simulink model "Assem1"  (R2017b)
settings: Solver=FixedStepAuto  StartTime=0.0  StopTime=40  FixedStep=0.01  RelTol=1e-3
model workspace: external: MATLAB File E:\RIC LAP Mo Phong\Robot4bac\Assem1_DataFile.m (data not in the file)
undefined symbols (not defined in the file or in its folder): smiData, X, Y, Z
libraries: sm_lib x29, nesl_utility x9, aerolibanimutils x1
settings Model: Creator=DELL  LastModifiedBy=DELL
settings OptimizationCC: BlockReduction=off

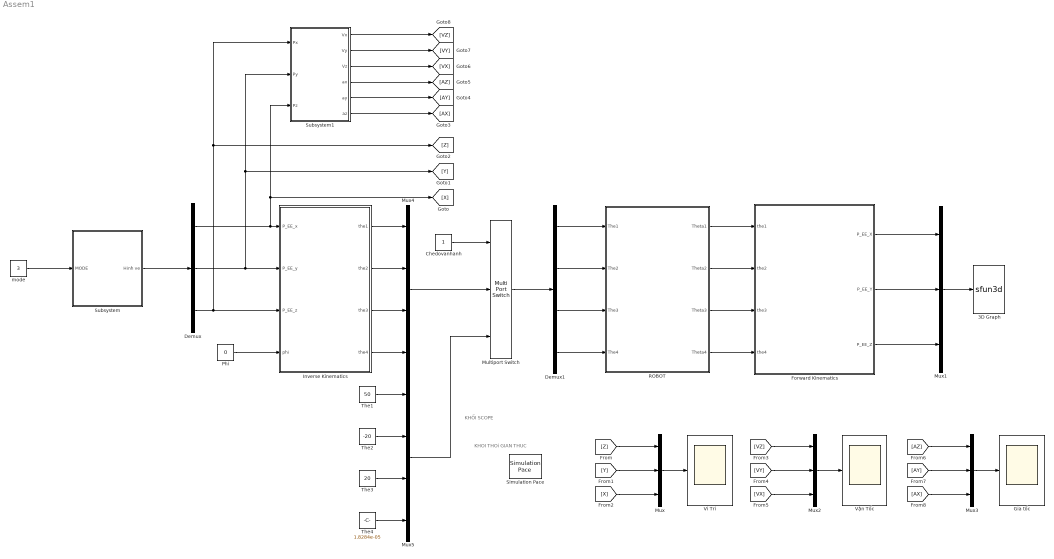
== system Assem1 ==
  note: KHOI THOi GIAN THUC
  note: KHỐI SCOPE
  3D Graph : S-Function  LoadFcn=if exist('sfun3d','file'), sfun3d([],[],[],'LoadBlock'); end  FunctionName=sfun3d  Parameters=ax,T,np,cp,gd,ls,mk,mx,hd,tb  SFunctionDeploymentMode=off  EnableBusSupport=off  mask(3D Graph){np=1, ax=[-500 1000 -500 1000 -500 1000], mx=1e4, T=0.01, cp=[3 2 1], gd=on, hd=off, tb=off, ls=:, mk=.}
      mask prompts: np "Number of moving points (lines)"; ax "Range: [xmin xmax  ymin ymax zmin zmax]"; mx "Max number of points in each line"; T "Sampling Time"; cp "Camera position (use [0 0 1] for 2D XY view)"; gd "Grid (on|off)"; hd "HeadMarkers (on|off)"; tb "Toolbar (on|off)"; ls "LineStyle"; mk "LineMarker"
      mask help:
      | This block plots the position of several points in the XYZ space. The input contains the coordinates of all the points (x1,y1,z1,x2,y2,z2,...).
      | The number of moving points (lines), the XYZ ranges, sampling time, camera position, and grid (among other things) can be set as mask parameters.
      settings: CopyFcn=if exist('sfun3d','file'), sfun3d([],[],[],'CopyBlock'); end  DeleteFcn=if exist('sfun3d','file'), sfun3d([],[],[],'DeleteBlock'); end  NameChangeFcn=if exist('sfun3d','file'), sfun3d([],[],[],'NameChange'); end
      mask Help:
      | This block plots the position of several points in the XYZ space. The input contains the coordinates of all the points (x1,y1,z1,x2,y2,z2,...).
      | The number of moving points (lines), the XYZ ranges, sampling time, camera position, and grid (among other things) can be set as mask parameters.
      mask TypeOptions ls: - | -- | : | -. | none
      mask TypeOptions mk: none | . | + | o | * | x | square | diamond | v | ^ | > | < | pentagram | hexagram
      mask Display: plot([.05 .95 .95 .05 .05],[.45 .45 .95 .95 .45], 0.5+cos(0:0.1:2*pi)*0.3,0.7+sin(0:0.1:2*pi)*0.2)
  Chedovanhanh : Constant
  Demux : Demux  Outputs=3
  Demux1 : Demux
  Forward Kinematics : MATLAB Function  TreatAsAtomicUnit=on
  Gia tốc : Scope
  Inverse Kinematics : MATLAB Function  TreatAsAtomicUnit=on
  Multiport Switch : MultiPortSwitch  Inputs=2
  Mux{,1..3} (4 alike) : Mux  Inputs=3
  Mux4 : Mux
  Mux5 : Mux
  Phi : Constant  Value=0
  "ROBOT " : Subsystem
  Simulation Pace : aerolibanimutils/Simulation Pace  SimulationPace=1  SleepMode=MATLAB Thread  OutputPaceError=off  SampleTime=0.01
  Subsystem : Subsystem
  Subsystem1 : Subsystem
  The1 : Constant  Value=50
  The2 : Constant  Value=-20
  The3 : Constant  Value=20
  The4 : Constant  Value=1.8284e-05
  Vi Tri : Scope
  Vận Tốc : Scope
  mode : Constant  Value=3
  wires:
  "ROBOT "/1(Theta1) -> Forward Kinematics/1(the1)
  "ROBOT "/2(Theta2) -> Forward Kinematics/2(the2)
  "ROBOT "/3(Theta3) -> Forward Kinematics/3(the3)
  "ROBOT "/4(Theta4) -> Forward Kinematics/4(the4)
  Chedovanhanh/1 -> Multiport Switch/1
  Mux4/1 -> Multiport Switch/2
  Multiport Switch/1 -> Demux1/1
  Inverse Kinematics/1(the1) -> Mux4/1
  Inverse Kinematics/2(the2) -> Mux4/2
  Inverse Kinematics/3(the3) -> Mux4/3
  Inverse Kinematics/4(the4) -> Mux4/4
  Demux1/1 -> "ROBOT "/1(The1)
  Demux1/2 -> "ROBOT "/2(The2)
  Demux1/3 -> "ROBOT "/3(The3)
  Demux1/4 -> "ROBOT "/4(The4)
  The4/1 -> Mux5/4
  The3/1 -> Mux5/3
  Mux5/1 -> Multiport Switch/3
  The1/1 -> Mux5/1
  The2/1 -> Mux5/2
  Subsystem/1(Hinh ve) -> Demux/1
  Subsystem1/3(Vz) -> [VX]
  Demux/3 -> Inverse Kinematics/3(P_EE_z), Subsystem1/1(Px), [Z]
  Subsystem1/6(az) -> [AX]
  Demux/2 -> Subsystem1/2(Py), [Y], Inverse Kinematics/2(P_EE_y)
  Subsystem1/2(Vy) -> [VY]
  Subsystem1/4(ax) -> [AZ]
  Subsystem1/5(ay) -> [AY]
  Subsystem1/1(Vx) -> [VZ]
  Demux/1 -> Subsystem1/3(Pz), [X], Inverse Kinematics/1(P_EE_x)
  [VY] -> Mux2/2
  Mux3/1 -> Gia tốc/1
  [VX] -> Mux2/3
  [AZ] -> Mux3/1
  [AY] -> Mux3/2
  Mux2/1 -> Vận Tốc/1
  [VZ] -> Mux2/1
  Mux/1 -> Vi Tri/1
  [Z] -> Mux/1
  [AX] -> Mux3/3
  [X] -> Mux/3
  [Y] -> Mux/2
  Mux1/1 -> 3D Graph/1
  Forward Kinematics/2(P_EE_Y) -> Mux1/2
  Forward Kinematics/3(P_EE_Z) -> Mux1/3
  Forward Kinematics/1(P_EE_X) -> Mux1/1
  mode/1 -> Subsystem/1(MODE)
  Phi/1 -> Inverse Kinematics/4(phi)

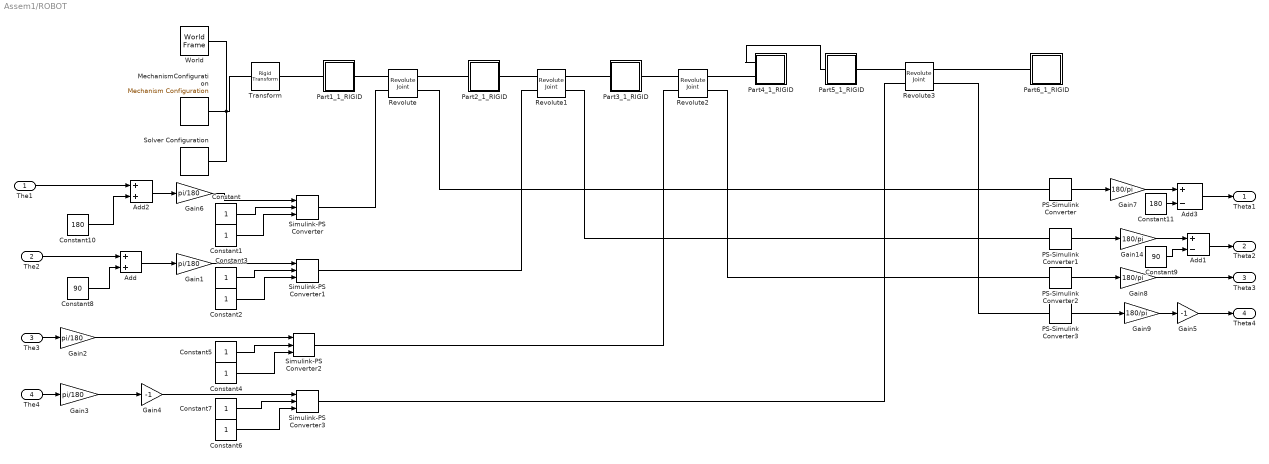
== system Assem1/ROBOT  ==
  The1 : Inport
  The2 : Inport  Port=2
  The3 : Inport  Port=3
  The4 : Inport  Port=4
  Add : Sum
  Add1 : Sum  Inputs=+-
  Add2 : Sum
  Add3 : Sum  Inputs=+-
  Constant{,1..7} (8 alike) : Constant
  Constant10 : Constant  Value=180
  Constant11 : Constant  Value=180
  Constant8 : Constant  Value=90
  Constant9 : Constant  Value=90
  Gain{1..3,6} (4 alike) : Gain  Gain=pi/180
  Gain{7..9,14} (4 alike) : Gain  Gain=180/pi
  Gain4 : Gain  Gain=-1
  Gain5 : Gain  Gain=-1
  MechanismConfiguration : sm_lib/Utilities/Mechanism Configuration  UniformGravity=Constant  GravityVector=[0 -9.80665 0]  GravityUnits=m/s^2  LinearizationDelta=0.001
  PS-Simulink Converter{,1..3} (4 alike) : nesl_utility/PS-Simulink Converter  PhysicalDomain=network_engine_domain  SubClassName=ps_output  LeftPortType=input  RightPortType=output  PseudoPeriodic=off  Frequencies=[]  Unit=1  AffineConversion=off
  Part1_1_RIGID : Subsystem
  Part2_1_RIGID : Subsystem
  Part3_1_RIGID : Subsystem
  Part4_1_RIGID : Subsystem
  Part5_1_RIGID : Subsystem
  Part6_1_RIGID : Subsystem
  Revolute : sm_lib/Joints/Revolute Joint  SenseConstraintForce=off  SenseConstraintForceX=off  SenseConstraintForceY=off  SenseConstraintForceZ=off  SenseConstraintTorque=off  SenseConstraintTorqueX=off  SenseConstraintTorqueY=off  SenseConstraintTorqueZ=off  SenseTotalForce=off  SenseTotalForceX=off  SenseTotalForceY=off  SenseTotalForceZ=off  SenseTotalTorque=off  SenseTotalTorqueX=off  SenseTotalTorqueY=off  SenseTotalTorqueZ=off  CompositeWrenchDir=FollowerOnBase  CompositeWrenchFrame=BaseFrame  EquilibriumPosition=0  EquilibriumPositionUnits=rad  SpringStiffness=0  SpringStiffnessUnits=N*m/rad  DampingCoefficient=0  DampingCoefficientUnits=N*m/(rad/s)  TorqueActuationMode=ComputedTorque  MotionActuationMode=InputMotion  SensePosition=on  SenseVelocity=off  SenseAcceleration=off  SenseTorqueForce=off  PositionTargetSpecify=on  PositionTargetPriority=Low  PositionTargetValue=smiData.RevoluteJoint(1).Rz.Pos  PositionTargetValueUnits=deg  VelocityTargetSpecify=off  VelocityTargetPriority=High  VelocityTargetValue=0  VelocityTargetValueUnits=deg/s
  Revolute1 : sm_lib/Joints/Revolute Joint  SenseConstraintForce=off  SenseConstraintForceX=off  SenseConstraintForceY=off  SenseConstraintForceZ=off  SenseConstraintTorque=off  SenseConstraintTorqueX=off  SenseConstraintTorqueY=off  SenseConstraintTorqueZ=off  SenseTotalForce=off  SenseTotalForceX=off  SenseTotalForceY=off  SenseTotalForceZ=off  SenseTotalTorque=off  SenseTotalTorqueX=off  SenseTotalTorqueY=off  SenseTotalTorqueZ=off  CompositeWrenchDir=FollowerOnBase  CompositeWrenchFrame=BaseFrame  EquilibriumPosition=0  EquilibriumPositionUnits=rad  SpringStiffness=0  SpringStiffnessUnits=N*m/rad  DampingCoefficient=0  DampingCoefficientUnits=N*m/(rad/s)  TorqueActuationMode=ComputedTorque  MotionActuationMode=InputMotion  SensePosition=on  SenseVelocity=off  SenseAcceleration=off  SenseTorqueForce=off  PositionTargetSpecify=on  PositionTargetPriority=Low  PositionTargetValue=smiData.RevoluteJoint(2).Rz.Pos  PositionTargetValueUnits=deg  VelocityTargetSpecify=off  VelocityTargetPriority=High  VelocityTargetValue=0  VelocityTargetValueUnits=deg/s
  Revolute2 : sm_lib/Joints/Revolute Joint  SenseConstraintForce=off  SenseConstraintForceX=off  SenseConstraintForceY=off  SenseConstraintForceZ=off  SenseConstraintTorque=off  SenseConstraintTorqueX=off  SenseConstraintTorqueY=off  SenseConstraintTorqueZ=off  SenseTotalForce=off  SenseTotalForceX=off  SenseTotalForceY=off  SenseTotalForceZ=off  SenseTotalTorque=off  SenseTotalTorqueX=off  SenseTotalTorqueY=off  SenseTotalTorqueZ=off  CompositeWrenchDir=FollowerOnBase  CompositeWrenchFrame=BaseFrame  EquilibriumPosition=0  EquilibriumPositionUnits=rad  SpringStiffness=0  SpringStiffnessUnits=N*m/rad  DampingCoefficient=0  DampingCoefficientUnits=N*m/(rad/s)  TorqueActuationMode=ComputedTorque  MotionActuationMode=InputMotion  SensePosition=on  SenseVelocity=off  SenseAcceleration=off  SenseTorqueForce=off  PositionTargetSpecify=on  PositionTargetPriority=Low  PositionTargetValue=smiData.RevoluteJoint(3).Rz.Pos  PositionTargetValueUnits=deg  VelocityTargetSpecify=off  VelocityTargetPriority=High  VelocityTargetValue=0  VelocityTargetValueUnits=deg/s
  Revolute3 : sm_lib/Joints/Revolute Joint  SenseConstraintForce=off  SenseConstraintForceX=off  SenseConstraintForceY=off  SenseConstraintForceZ=off  SenseConstraintTorque=off  SenseConstraintTorqueX=off  SenseConstraintTorqueY=off  SenseConstraintTorqueZ=off  SenseTotalForce=off  SenseTotalForceX=off  SenseTotalForceY=off  SenseTotalForceZ=off  SenseTotalTorque=off  SenseTotalTorqueX=off  SenseTotalTorqueY=off  SenseTotalTorqueZ=off  CompositeWrenchDir=FollowerOnBase  CompositeWrenchFrame=BaseFrame  EquilibriumPosition=0  EquilibriumPositionUnits=rad  SpringStiffness=0  SpringStiffnessUnits=N*m/rad  DampingCoefficient=0  DampingCoefficientUnits=N*m/(rad/s)  TorqueActuationMode=ComputedTorque  MotionActuationMode=InputMotion  SensePosition=on  SenseVelocity=off  SenseAcceleration=off  SenseTorqueForce=off  PositionTargetSpecify=on  PositionTargetPriority=Low  PositionTargetValue=smiData.RevoluteJoint(4).Rz.Pos  PositionTargetValueUnits=deg  VelocityTargetSpecify=off  VelocityTargetPriority=High  VelocityTargetValue=0  VelocityTargetValueUnits=deg/s
  Simulink-PS Converter{,1..3} (4 alike) : nesl_utility/Simulink-PS Converter  PhysicalDomain=network_engine_domain  SubClassName=ps_input  LeftPortType=input  RightPortType=output  PseudoPeriodic=off  Frequencies=[]  NoiseDistribution=none  NoiseParameters=[]  Unit=1  AffineConversion=off  FilteringAndDerivatives=provide  SimscapeFilterOrder=1  InputFilterTimeConstant=0.001  UdotUserProvided=2
  Solver Configuration : nesl_utility/Solver Configuration  PhysicalDomain=network_engine_domain  SubClassName=solver  LeftPortType=input  RightPortType=generic  Accelerate=off  Tones=[]  Harmonics=[]  SimulateNoise=off  Profile=off  UseLocalSampling=off  EnableSwitchedLinearOptims=on  FrequencyDomain=off  UseCCode=off  RelTol=0.001  AbsTol=1e-06  MinStep=1e-09  ToWorkspace=off  RevertToSquareIcSolve=off  NumHomotopyIterations=100  PhasorMode=off  PhasorModeNumHarmonics=1  DoDC=off  ResidualTolerance=1e-09  UseLocalSolver=off  LocalSolverChoice=NE_BACKWARD_EULER_ADVANCER  LocalSolverSampleTime=0.001  DoFixedCost=off  MaxNonlinIter=3  MaxModeIter=2  LinearAlgebra=Sparse  DelaysMemoryBudget=1024  AutomaticFiltering=on  FilteringTimeConstant=0.001
  Transform : sm_lib/Frames and Transforms/Rigid Transform  TranslationMethod=Cartesian  TranslationStandardOffset=0  TranslationLengthUnit=mm  TranslationStandardAxis=+Z  TranslationCartesianOffset=smiData.RigidTransform(11).translation  TranslationROffset=0  TranslationROffsetUnits=m  TranslationZOffset=0  TranslationZOffsetUnits=m  TranslationThetaOffset=0  TranslationThetaOffsetUnits=deg  RotationMethod=ArbitraryAxis  RotationAngleUnits=rad  RotationStandardAxis=+Z  RotationAngle=smiData.RigidTransform(11).angle  RotationArbitraryAxis=smiData.RigidTransform(11).axis  FollAlignAxisA=+X  BaseAlignAxisA=+Y  FollAlignAxisB=+Y  BaseAlignAxisB=+Z  RotationSequenceAxes=FollowerAxes  RotationSequence=XYX  RotationSequenceAngles=[0 0 0]  RotationSequenceAnglesUnits=deg  RotationMatrix=[1 0 0; 0 1 0; 0 0 1]
  World : sm_lib/Frames and Transforms/World Frame
  Theta1 : Outport
  Theta2 : Outport  Port=2
  Theta3 : Outport  Port=3
  Theta4 : Outport  Port=4
  wires:
  PS-Simulink Converter/1 -> Gain7/1
  PS-Simulink Converter3/1 -> Gain9/1
  Gain8/1 -> Theta3/1
  PS-Simulink Converter2/1 -> Gain8/1
  PS-Simulink Converter1/1 -> Gain14/1
  Gain2/1 -> Simulink-PS Converter2/1
  The3/1 -> Gain2/1
  Gain1/1 -> Simulink-PS Converter1/1
  Gain3/1 -> Gain4/1
  The4/1 -> Gain3/1
  Constant/1 -> Simulink-PS Converter/2
  Constant1/1 -> Simulink-PS Converter/3
  Constant3/1 -> Simulink-PS Converter1/2
  Constant2/1 -> Simulink-PS Converter1/3
  Constant5/1 -> Simulink-PS Converter2/2
  Constant4/1 -> Simulink-PS Converter2/3
  Constant7/1 -> Simulink-PS Converter3/2
  Constant6/1 -> Simulink-PS Converter3/3
  The2/1 -> Add/1
  Add/1 -> Gain1/1
  Constant8/1 -> Add/2
  Gain4/1 -> Simulink-PS Converter3/1
  Gain5/1 -> Theta4/1
  Gain9/1 -> Gain5/1
  Gain14/1 -> Add1/1
  Add1/1 -> Theta2/1
  Constant9/1 -> Add1/2
  Add2/1 -> Gain6/1
  Constant10/1 -> Add2/2
  Gain6/1 -> Simulink-PS Converter/1
  The1/1 -> Add2/1
  Gain7/1 -> Add3/1
  Add3/1 -> Theta1/1
  Constant11/1 -> Add3/2
  connections:
  PS-Simulink Converter/LConn1 -- Revolute/RConn2
  PS-Simulink Converter2/LConn1 -- Revolute2/RConn2
  PS-Simulink Converter1/LConn1 -- Revolute1/RConn2
  PS-Simulink Converter3/LConn1 -- Revolute3/RConn2
  Part2_1_RIGID/RConn1 -- Revolute1/LConn1
  Part2_1_RIGID/LConn1 -- Revolute/RConn1
  Part1_1_RIGID/LConn1 -- Transform/RConn1
  Part6_1_RIGID/LConn1 -- Revolute3/RConn1
  Part3_1_RIGID/LConn1 -- Revolute1/RConn1
  Part4_1_RIGID/LConn2 -- Revolute2/RConn1
  Part5_1_RIGID/RConn1 -- Revolute3/LConn1
  Part4_1_RIGID/LConn1 -- Part5_1_RIGID/LConn1
  Part3_1_RIGID/RConn1 -- Revolute2/LConn1
  Part1_1_RIGID/RConn1 -- Revolute/LConn1
  Transform/LConn1 -- MechanismConfiguration/RConn1 -- Solver Configuration/RConn1 -- World/RConn1
  Simulink-PS Converter/RConn1 -- Revolute/LConn2
  Simulink-PS Converter1/RConn1 -- Revolute1/LConn2
  Simulink-PS Converter3/RConn1 -- Revolute3/LConn2
  Simulink-PS Converter2/RConn1 -- Revolute2/LConn2

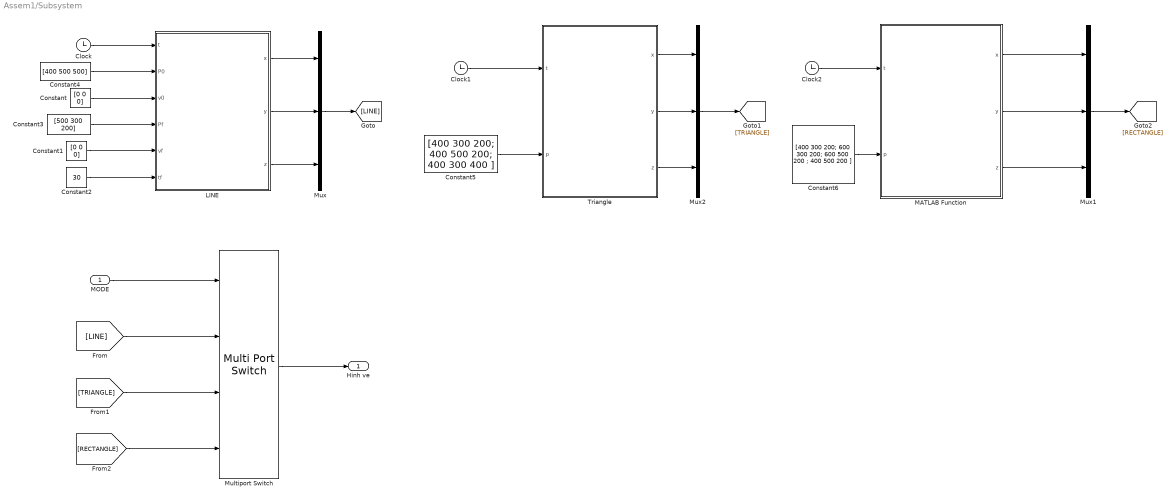
== system Assem1/Subsystem ==
  MODE : Inport
  Clock : Clock
      settings: Decimation=30
  Clock1 : Clock
      settings: Decimation=30
  Clock2 : Clock
      settings: Decimation=40
  Constant : Constant  Value=[0 0 0]
  Constant1 : Constant  Value=[0 0 0]
  Constant2 : Constant  Value=30
  Constant3 : Constant  Value=[500 300 200]
  Constant4 : Constant  Value=[400 500 500]
  Constant5 : Constant  Value="[400 300 200; 400 500 200; 400 300 400  ]"
  Constant6 : Constant  Value=[400 300 200; 600 300 200; 600 500 200 ; 400 500 200 ]
  "LINE   " : MATLAB Function  TreatAsAtomicUnit=on
  MATLAB Function : MATLAB Function  TreatAsAtomicUnit=on
  Multiport Switch : MultiPortSwitch
  Mux : Mux  Inputs=3
  Mux1 : Mux  Inputs=3
  Mux2 : Mux  Inputs=3
  Triangle : MATLAB Function  TreatAsAtomicUnit=on
  Hinh ve : Outport
  wires:
  Clock1/1 -> Triangle/1(t)
  Constant4/1 -> "LINE   "/2(P0)
  Constant3/1 -> "LINE   "/4(Pf)
  Clock/1 -> "LINE   "/1(t)
  Constant2/1 -> "LINE   "/6(tf)
  Constant/1 -> "LINE   "/3(v0)
  Constant1/1 -> "LINE   "/5(vf)
  MODE/1 -> Multiport Switch/1
  "LINE   "/1(x) -> Mux/1
  "LINE   "/2(y) -> Mux/2
  "LINE   "/3(z) -> Mux/3
  Mux/1 -> [LINE]
  [LINE] -> Multiport Switch/2
  [TRIANGLE] -> Multiport Switch/3
  [RECTANGLE] -> Multiport Switch/4
  Triangle/1(x) -> Mux2/1
  Triangle/2(y) -> Mux2/2
  Mux2/1 -> [TRIANGLE]
  Triangle/3(z) -> Mux2/3
  Constant5/1 -> Triangle/2(p)
  Mux1/1 -> [RECTANGLE]
  MATLAB Function/1(x) -> Mux1/1
  MATLAB Function/2(y) -> Mux1/2
  MATLAB Function/3(z) -> Mux1/3
  Clock2/1 -> MATLAB Function/1(t)
  Constant6/1 -> MATLAB Function/2(p)
  Multiport Switch/1 -> Hinh ve/1

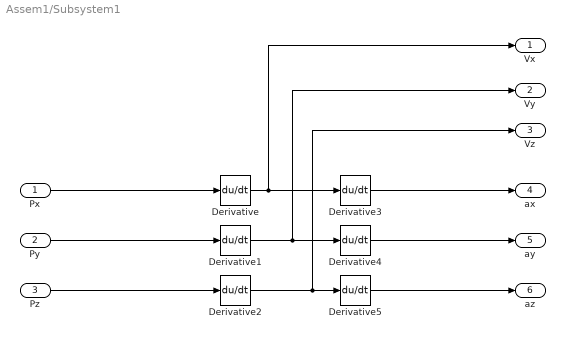
== system Assem1/Subsystem1 ==
  Px : Inport
  Py : Inport  Port=2
  Pz : Inport  Port=3
  Derivative{,1..5} (6 alike) : Derivative
  Vx : Outport
  Vy : Outport  Port=2
  Vz : Outport  Port=3
  ax : Outport  Port=4
  ay : Outport  Port=5
  az : Outport  Port=6
  wires:
  Derivative4/1 -> ay/1
  Px/1 -> Derivative/1
  Py/1 -> Derivative1/1
  Pz/1 -> Derivative2/1
  Derivative5/1 -> az/1
  Derivative2/1 -> Vz/1, Derivative5/1
  Derivative/1 -> Vx/1, Derivative3/1
  Derivative1/1 -> Vy/1, Derivative4/1
  Derivative3/1 -> ax/1

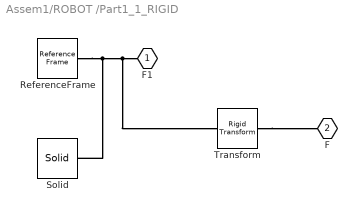
== system Assem1/ROBOT /Part1_1_RIGID ==
  ReferenceFrame : sm_lib/Frames and Transforms/Reference Frame
  Solid : sm_lib/Body Elements/Solid  InertiaType=Custom  Mass=smiData.Solid(4).mass  MassUnits=kg  CenterOfMass=smiData.Solid(4).CoM  CenterOfMassUnits=mm  MomentsOfInertia=smiData.Solid(4).MoI  MomentsOfInertiaUnits=kg*mm^2  ProductsOfInertia=smiData.Solid(4).PoI  ProductsOfInertiaUnits=kg*mm^2  DensityBased=on  Density=1000  DensityUnits=kg/m^3  DoExposeReferenceFrame=on  SerializedFrames=<Frames/>  GraphicType=FromGeometry  MarkerShape=Sphere  MarkerSize=10  GraphicVisPropType=SimpleVisualProperties  GraphicDiffuseColor=smiData.Solid(4).color  GraphicSpecularColor=[0.5 0.5 0.5 1.0]  GraphicAmbientColor=[0.15 0.15 0.15 1.0]  GraphicEmissiveColor=[0.0 0.0 0.0 1.0]  GraphicShininess=75  GraphicOpacity=smiData.Solid(4).opacity  GeometryShape=FromFile  RectangleSize=[1 1]  RectangleSizeUnits=m  BrickDimensions=[1 1 1]  BrickDimensionUnits=m  CylinderRadius=1  CylinderRadiusUnits=m  CylinderLength=1  CylinderLengthUnits=m  SphereRadius=1  SphereRadiusUnits=m  EllipsoidRadii=[1 1 1]  EllipsoidRadiiUnits=m  ExtrusionCrossSection=[1 1; -1 1; -1 -1; 1 -1]  ExtrusionCrossSectionUnits=m  ExtrusionLength=1  ExtrusionLengthUnits=m  PolygonNumSides=3  PolygonOuterRadius=1  PolygonOuterRadiusUnits=m  ExtGeomFileType=STEP  ExtGeomFileName=Part1_Default_sldprt.STEP  ExtGeomFileUnits=m  RevolutionCrossSection=[1 1; 1 -1; 2 -1; 2 1]  RevolutionCrossSectionUnits=m  RevolutionExtent=Full  RevolutionAngle=180  RevolutionAngleUnits=deg
  Transform : sm_lib/Frames and Transforms/Rigid Transform  TranslationMethod=Cartesian  TranslationStandardOffset=0  TranslationLengthUnit=mm  TranslationStandardAxis=+Z  TranslationCartesianOffset=smiData.RigidTransform(1).translation  TranslationROffset=0  TranslationROffsetUnits=m  TranslationZOffset=0  TranslationZOffsetUnits=m  TranslationThetaOffset=0  TranslationThetaOffsetUnits=deg  RotationMethod=ArbitraryAxis  RotationAngleUnits=rad  RotationStandardAxis=+Z  RotationAngle=smiData.RigidTransform(1).angle  RotationArbitraryAxis=smiData.RigidTransform(1).axis  FollAlignAxisA=+X  BaseAlignAxisA=+Y  FollAlignAxisB=+Y  BaseAlignAxisB=+Z  RotationSequenceAxes=FollowerAxes  RotationSequence=XYX  RotationSequenceAngles=[0 0 0]  RotationSequenceAnglesUnits=deg  RotationMatrix=[1 0 0; 0 1 0; 0 0 1]
  F1 : PMIOPort  Port=1  Side=Left
  F : PMIOPort  Port=2  Side=Right
  connections:
  Solid/RConn1 -- ReferenceFrame/RConn1 -- Transform/LConn1 -- F1/RConn1
  Transform/RConn1 -- F/RConn1

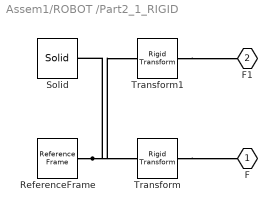
== system Assem1/ROBOT /Part2_1_RIGID ==
  ReferenceFrame : sm_lib/Frames and Transforms/Reference Frame
  Solid : sm_lib/Body Elements/Solid  InertiaType=Custom  Mass=smiData.Solid(2).mass  MassUnits=kg  CenterOfMass=smiData.Solid(2).CoM  CenterOfMassUnits=mm  MomentsOfInertia=smiData.Solid(2).MoI  MomentsOfInertiaUnits=kg*mm^2  ProductsOfInertia=smiData.Solid(2).PoI  ProductsOfInertiaUnits=kg*mm^2  DensityBased=on  Density=1000  DensityUnits=kg/m^3  DoExposeReferenceFrame=on  SerializedFrames=<Frames/>  GraphicType=FromGeometry  MarkerShape=Sphere  MarkerSize=10  GraphicVisPropType=SimpleVisualProperties  GraphicDiffuseColor=smiData.Solid(2).color  GraphicSpecularColor=[0.5 0.5 0.5 1.0]  GraphicAmbientColor=[0.15 0.15 0.15 1.0]  GraphicEmissiveColor=[0.0 0.0 0.0 1.0]  GraphicShininess=75  GraphicOpacity=smiData.Solid(2).opacity  GeometryShape=FromFile  RectangleSize=[1 1]  RectangleSizeUnits=m  BrickDimensions=[1 1 1]  BrickDimensionUnits=m  CylinderRadius=1  CylinderRadiusUnits=m  CylinderLength=1  CylinderLengthUnits=m  SphereRadius=1  SphereRadiusUnits=m  EllipsoidRadii=[1 1 1]  EllipsoidRadiiUnits=m  ExtrusionCrossSection=[1 1; -1 1; -1 -1; 1 -1]  ExtrusionCrossSectionUnits=m  ExtrusionLength=1  ExtrusionLengthUnits=m  PolygonNumSides=3  PolygonOuterRadius=1  PolygonOuterRadiusUnits=m  ExtGeomFileType=STEP  ExtGeomFileName=Part2_Default_sldprt.STEP  ExtGeomFileUnits=m  RevolutionCrossSection=[1 1; 1 -1; 2 -1; 2 1]  RevolutionCrossSectionUnits=m  RevolutionExtent=Full  RevolutionAngle=180  RevolutionAngleUnits=deg
  Transform : sm_lib/Frames and Transforms/Rigid Transform  TranslationMethod=Cartesian  TranslationStandardOffset=0  TranslationLengthUnit=mm  TranslationStandardAxis=+Z  TranslationCartesianOffset=smiData.RigidTransform(2).translation  TranslationROffset=0  TranslationROffsetUnits=m  TranslationZOffset=0  TranslationZOffsetUnits=m  TranslationThetaOffset=0  TranslationThetaOffsetUnits=deg  RotationMethod=ArbitraryAxis  RotationAngleUnits=rad  RotationStandardAxis=+Z  RotationAngle=smiData.RigidTransform(2).angle  RotationArbitraryAxis=smiData.RigidTransform(2).axis  FollAlignAxisA=+X  BaseAlignAxisA=+Y  FollAlignAxisB=+Y  BaseAlignAxisB=+Z  RotationSequenceAxes=FollowerAxes  RotationSequence=XYX  RotationSequenceAngles=[0 0 0]  RotationSequenceAnglesUnits=deg  RotationMatrix=[1 0 0; 0 1 0; 0 0 1]
  Transform1 : sm_lib/Frames and Transforms/Rigid Transform  TranslationMethod=Cartesian  TranslationStandardOffset=0  TranslationLengthUnit=mm  TranslationStandardAxis=+Z  TranslationCartesianOffset=smiData.RigidTransform(3).translation  TranslationROffset=0  TranslationROffsetUnits=m  TranslationZOffset=0  TranslationZOffsetUnits=m  TranslationThetaOffset=0  TranslationThetaOffsetUnits=deg  RotationMethod=ArbitraryAxis  RotationAngleUnits=rad  RotationStandardAxis=+Z  RotationAngle=smiData.RigidTransform(3).angle  RotationArbitraryAxis=smiData.RigidTransform(3).axis  FollAlignAxisA=+X  BaseAlignAxisA=+Y  FollAlignAxisB=+Y  BaseAlignAxisB=+Z  RotationSequenceAxes=FollowerAxes  RotationSequence=XYX  RotationSequenceAngles=[0 0 0]  RotationSequenceAnglesUnits=deg  RotationMatrix=[1 0 0; 0 1 0; 0 0 1]
  F : PMIOPort  Port=1  Side=Left
  F1 : PMIOPort  Port=2  Side=Right
  connections:
  Solid/RConn1 -- ReferenceFrame/RConn1 -- Transform/LConn1 -- Transform1/LConn1
  Transform/RConn1 -- F/RConn1
  Transform1/RConn1 -- F1/RConn1

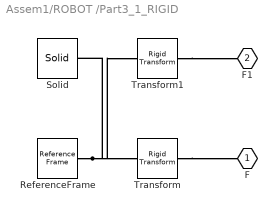
== system Assem1/ROBOT /Part3_1_RIGID ==
  ReferenceFrame : sm_lib/Frames and Transforms/Reference Frame
  Solid : sm_lib/Body Elements/Solid  InertiaType=Custom  Mass=smiData.Solid(3).mass  MassUnits=kg  CenterOfMass=smiData.Solid(3).CoM  CenterOfMassUnits=mm  MomentsOfInertia=smiData.Solid(3).MoI  MomentsOfInertiaUnits=kg*mm^2  ProductsOfInertia=smiData.Solid(3).PoI  ProductsOfInertiaUnits=kg*mm^2  DensityBased=on  Density=1000  DensityUnits=kg/m^3  DoExposeReferenceFrame=on  SerializedFrames=<Frames/>  GraphicType=FromGeometry  MarkerShape=Sphere  MarkerSize=10  GraphicVisPropType=SimpleVisualProperties  GraphicDiffuseColor=smiData.Solid(3).color  GraphicSpecularColor=[0.5 0.5 0.5 1.0]  GraphicAmbientColor=[0.15 0.15 0.15 1.0]  GraphicEmissiveColor=[0.0 0.0 0.0 1.0]  GraphicShininess=75  GraphicOpacity=smiData.Solid(3).opacity  GeometryShape=FromFile  RectangleSize=[1 1]  RectangleSizeUnits=m  BrickDimensions=[1 1 1]  BrickDimensionUnits=m  CylinderRadius=1  CylinderRadiusUnits=m  CylinderLength=1  CylinderLengthUnits=m  SphereRadius=1  SphereRadiusUnits=m  EllipsoidRadii=[1 1 1]  EllipsoidRadiiUnits=m  ExtrusionCrossSection=[1 1; -1 1; -1 -1; 1 -1]  ExtrusionCrossSectionUnits=m  ExtrusionLength=1  ExtrusionLengthUnits=m  PolygonNumSides=3  PolygonOuterRadius=1  PolygonOuterRadiusUnits=m  ExtGeomFileType=STEP  ExtGeomFileName=Part3_Default_sldprt.STEP  ExtGeomFileUnits=m  RevolutionCrossSection=[1 1; 1 -1; 2 -1; 2 1]  RevolutionCrossSectionUnits=m  RevolutionExtent=Full  RevolutionAngle=180  RevolutionAngleUnits=deg
  Transform : sm_lib/Frames and Transforms/Rigid Transform  TranslationMethod=Cartesian  TranslationStandardOffset=0  TranslationLengthUnit=mm  TranslationStandardAxis=+Z  TranslationCartesianOffset=smiData.RigidTransform(4).translation  TranslationROffset=0  TranslationROffsetUnits=m  TranslationZOffset=0  TranslationZOffsetUnits=m  TranslationThetaOffset=0  TranslationThetaOffsetUnits=deg  RotationMethod=ArbitraryAxis  RotationAngleUnits=rad  RotationStandardAxis=+Z  RotationAngle=smiData.RigidTransform(4).angle  RotationArbitraryAxis=smiData.RigidTransform(4).axis  FollAlignAxisA=+X  BaseAlignAxisA=+Y  FollAlignAxisB=+Y  BaseAlignAxisB=+Z  RotationSequenceAxes=FollowerAxes  RotationSequence=XYX  RotationSequenceAngles=[0 0 0]  RotationSequenceAnglesUnits=deg  RotationMatrix=[1 0 0; 0 1 0; 0 0 1]
  Transform1 : sm_lib/Frames and Transforms/Rigid Transform  TranslationMethod=Cartesian  TranslationStandardOffset=0  TranslationLengthUnit=mm  TranslationStandardAxis=+Z  TranslationCartesianOffset=smiData.RigidTransform(5).translation  TranslationROffset=0  TranslationROffsetUnits=m  TranslationZOffset=0  TranslationZOffsetUnits=m  TranslationThetaOffset=0  TranslationThetaOffsetUnits=deg  RotationMethod=ArbitraryAxis  RotationAngleUnits=rad  RotationStandardAxis=+Z  RotationAngle=smiData.RigidTransform(5).angle  RotationArbitraryAxis=smiData.RigidTransform(5).axis  FollAlignAxisA=+X  BaseAlignAxisA=+Y  FollAlignAxisB=+Y  BaseAlignAxisB=+Z  RotationSequenceAxes=FollowerAxes  RotationSequence=XYX  RotationSequenceAngles=[0 0 0]  RotationSequenceAnglesUnits=deg  RotationMatrix=[1 0 0; 0 1 0; 0 0 1]
  F : PMIOPort  Port=1  Side=Left
  F1 : PMIOPort  Port=2  Side=Right
  connections:
  Solid/RConn1 -- ReferenceFrame/RConn1 -- Transform/LConn1 -- Transform1/LConn1
  Transform/RConn1 -- F/RConn1
  Transform1/RConn1 -- F1/RConn1

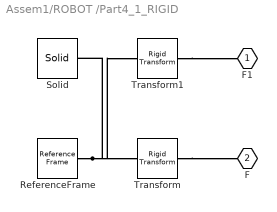
== system Assem1/ROBOT /Part4_1_RIGID ==
  ReferenceFrame : sm_lib/Frames and Transforms/Reference Frame
  Solid : sm_lib/Body Elements/Solid  InertiaType=Custom  Mass=smiData.Solid(1).mass  MassUnits=kg  CenterOfMass=smiData.Solid(1).CoM  CenterOfMassUnits=mm  MomentsOfInertia=smiData.Solid(1).MoI  MomentsOfInertiaUnits=kg*mm^2  ProductsOfInertia=smiData.Solid(1).PoI  ProductsOfInertiaUnits=kg*mm^2  DensityBased=on  Density=1000  DensityUnits=kg/m^3  DoExposeReferenceFrame=on  SerializedFrames=<Frames/>  GraphicType=FromGeometry  MarkerShape=Sphere  MarkerSize=10  GraphicVisPropType=SimpleVisualProperties  GraphicDiffuseColor=smiData.Solid(1).color  GraphicSpecularColor=[0.5 0.5 0.5 1.0]  GraphicAmbientColor=[0.15 0.15 0.15 1.0]  GraphicEmissiveColor=[0.0 0.0 0.0 1.0]  GraphicShininess=75  GraphicOpacity=smiData.Solid(1).opacity  GeometryShape=FromFile  RectangleSize=[1 1]  RectangleSizeUnits=m  BrickDimensions=[1 1 1]  BrickDimensionUnits=m  CylinderRadius=1  CylinderRadiusUnits=m  CylinderLength=1  CylinderLengthUnits=m  SphereRadius=1  SphereRadiusUnits=m  EllipsoidRadii=[1 1 1]  EllipsoidRadiiUnits=m  ExtrusionCrossSection=[1 1; -1 1; -1 -1; 1 -1]  ExtrusionCrossSectionUnits=m  ExtrusionLength=1  ExtrusionLengthUnits=m  PolygonNumSides=3  PolygonOuterRadius=1  PolygonOuterRadiusUnits=m  ExtGeomFileType=STEP  ExtGeomFileName=Part4_Default_sldprt.STEP  ExtGeomFileUnits=m  RevolutionCrossSection=[1 1; 1 -1; 2 -1; 2 1]  RevolutionCrossSectionUnits=m  RevolutionExtent=Full  RevolutionAngle=180  RevolutionAngleUnits=deg
  Transform : sm_lib/Frames and Transforms/Rigid Transform  TranslationMethod=Cartesian  TranslationStandardOffset=0  TranslationLengthUnit=mm  TranslationStandardAxis=+Z  TranslationCartesianOffset=smiData.RigidTransform(6).translation  TranslationROffset=0  TranslationROffsetUnits=m  TranslationZOffset=0  TranslationZOffsetUnits=m  TranslationThetaOffset=0  TranslationThetaOffsetUnits=deg  RotationMethod=ArbitraryAxis  RotationAngleUnits=rad  RotationStandardAxis=+Z  RotationAngle=smiData.RigidTransform(6).angle  RotationArbitraryAxis=smiData.RigidTransform(6).axis  FollAlignAxisA=+X  BaseAlignAxisA=+Y  FollAlignAxisB=+Y  BaseAlignAxisB=+Z  RotationSequenceAxes=FollowerAxes  RotationSequence=XYX  RotationSequenceAngles=[0 0 0]  RotationSequenceAnglesUnits=deg  RotationMatrix=[1 0 0; 0 1 0; 0 0 1]
  Transform1 : sm_lib/Frames and Transforms/Rigid Transform  TranslationMethod=Cartesian  TranslationStandardOffset=0  TranslationLengthUnit=mm  TranslationStandardAxis=+Z  TranslationCartesianOffset=smiData.RigidTransform(7).translation  TranslationROffset=0  TranslationROffsetUnits=m  TranslationZOffset=0  TranslationZOffsetUnits=m  TranslationThetaOffset=0  TranslationThetaOffsetUnits=deg  RotationMethod=ArbitraryAxis  RotationAngleUnits=rad  RotationStandardAxis=+Z  RotationAngle=smiData.RigidTransform(7).angle  RotationArbitraryAxis=smiData.RigidTransform(7).axis  FollAlignAxisA=+X  BaseAlignAxisA=+Y  FollAlignAxisB=+Y  BaseAlignAxisB=+Z  RotationSequenceAxes=FollowerAxes  RotationSequence=XYX  RotationSequenceAngles=[0 0 0]  RotationSequenceAnglesUnits=deg  RotationMatrix=[1 0 0; 0 1 0; 0 0 1]
  F1 : PMIOPort  Port=1  Side=Left
  F : PMIOPort  Port=2  Side=Left
  connections:
  Solid/RConn1 -- ReferenceFrame/RConn1 -- Transform/LConn1 -- Transform1/LConn1
  Transform/RConn1 -- F/RConn1
  Transform1/RConn1 -- F1/RConn1

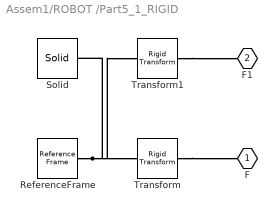
== system Assem1/ROBOT /Part5_1_RIGID ==
  ReferenceFrame : sm_lib/Frames and Transforms/Reference Frame
  Solid : sm_lib/Body Elements/Solid  InertiaType=Custom  Mass=smiData.Solid(6).mass  MassUnits=kg  CenterOfMass=smiData.Solid(6).CoM  CenterOfMassUnits=mm  MomentsOfInertia=smiData.Solid(6).MoI  MomentsOfInertiaUnits=kg*mm^2  ProductsOfInertia=smiData.Solid(6).PoI  ProductsOfInertiaUnits=kg*mm^2  DensityBased=on  Density=1000  DensityUnits=kg/m^3  DoExposeReferenceFrame=on  SerializedFrames=<Frames/>  GraphicType=FromGeometry  MarkerShape=Sphere  MarkerSize=10  GraphicVisPropType=SimpleVisualProperties  GraphicDiffuseColor=smiData.Solid(6).color  GraphicSpecularColor=[0.5 0.5 0.5 1.0]  GraphicAmbientColor=[0.15 0.15 0.15 1.0]  GraphicEmissiveColor=[0.0 0.0 0.0 1.0]  GraphicShininess=75  GraphicOpacity=smiData.Solid(6).opacity  GeometryShape=FromFile  RectangleSize=[1 1]  RectangleSizeUnits=m  BrickDimensions=[1 1 1]  BrickDimensionUnits=m  CylinderRadius=1  CylinderRadiusUnits=m  CylinderLength=1  CylinderLengthUnits=m  SphereRadius=1  SphereRadiusUnits=m  EllipsoidRadii=[1 1 1]  EllipsoidRadiiUnits=m  ExtrusionCrossSection=[1 1; -1 1; -1 -1; 1 -1]  ExtrusionCrossSectionUnits=m  ExtrusionLength=1  ExtrusionLengthUnits=m  PolygonNumSides=3  PolygonOuterRadius=1  PolygonOuterRadiusUnits=m  ExtGeomFileType=STEP  ExtGeomFileName=Part5_Default_sldprt.STEP  ExtGeomFileUnits=m  RevolutionCrossSection=[1 1; 1 -1; 2 -1; 2 1]  RevolutionCrossSectionUnits=m  RevolutionExtent=Full  RevolutionAngle=180  RevolutionAngleUnits=deg
  Transform : sm_lib/Frames and Transforms/Rigid Transform  TranslationMethod=Cartesian  TranslationStandardOffset=0  TranslationLengthUnit=mm  TranslationStandardAxis=+Z  TranslationCartesianOffset=smiData.RigidTransform(8).translation  TranslationROffset=0  TranslationROffsetUnits=m  TranslationZOffset=0  TranslationZOffsetUnits=m  TranslationThetaOffset=0  TranslationThetaOffsetUnits=deg  RotationMethod=ArbitraryAxis  RotationAngleUnits=rad  RotationStandardAxis=+Z  RotationAngle=smiData.RigidTransform(8).angle  RotationArbitraryAxis=smiData.RigidTransform(8).axis  FollAlignAxisA=+X  BaseAlignAxisA=+Y  FollAlignAxisB=+Y  BaseAlignAxisB=+Z  RotationSequenceAxes=FollowerAxes  RotationSequence=XYX  RotationSequenceAngles=[0 0 0]  RotationSequenceAnglesUnits=deg  RotationMatrix=[1 0 0; 0 1 0; 0 0 1]
  Transform1 : sm_lib/Frames and Transforms/Rigid Transform  TranslationMethod=Cartesian  TranslationStandardOffset=0  TranslationLengthUnit=mm  TranslationStandardAxis=+Z  TranslationCartesianOffset=smiData.RigidTransform(9).translation  TranslationROffset=0  TranslationROffsetUnits=m  TranslationZOffset=0  TranslationZOffsetUnits=m  TranslationThetaOffset=0  TranslationThetaOffsetUnits=deg  RotationMethod=ArbitraryAxis  RotationAngleUnits=rad  RotationStandardAxis=+Z  RotationAngle=smiData.RigidTransform(9).angle  RotationArbitraryAxis=smiData.RigidTransform(9).axis  FollAlignAxisA=+X  BaseAlignAxisA=+Y  FollAlignAxisB=+Y  BaseAlignAxisB=+Z  RotationSequenceAxes=FollowerAxes  RotationSequence=XYX  RotationSequenceAngles=[0 0 0]  RotationSequenceAnglesUnits=deg  RotationMatrix=[1 0 0; 0 1 0; 0 0 1]
  F : PMIOPort  Port=1  Side=Left
  F1 : PMIOPort  Port=2  Side=Right
  connections:
  Solid/RConn1 -- ReferenceFrame/RConn1 -- Transform/LConn1 -- Transform1/LConn1
  Transform/RConn1 -- F/RConn1
  Transform1/RConn1 -- F1/RConn1

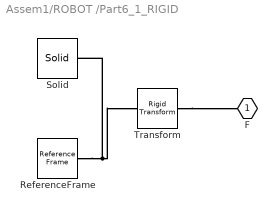
== system Assem1/ROBOT /Part6_1_RIGID ==
  ReferenceFrame : sm_lib/Frames and Transforms/Reference Frame
  Solid : sm_lib/Body Elements/Solid  InertiaType=Custom  Mass=smiData.Solid(5).mass  MassUnits=kg  CenterOfMass=smiData.Solid(5).CoM  CenterOfMassUnits=mm  MomentsOfInertia=smiData.Solid(5).MoI  MomentsOfInertiaUnits=kg*mm^2  ProductsOfInertia=smiData.Solid(5).PoI  ProductsOfInertiaUnits=kg*mm^2  DensityBased=on  Density=1000  DensityUnits=kg/m^3  DoExposeReferenceFrame=on  SerializedFrames=<Frames/>  GraphicType=FromGeometry  MarkerShape=Sphere  MarkerSize=10  GraphicVisPropType=SimpleVisualProperties  GraphicDiffuseColor=smiData.Solid(5).color  GraphicSpecularColor=[0.5 0.5 0.5 1.0]  GraphicAmbientColor=[0.15 0.15 0.15 1.0]  GraphicEmissiveColor=[0.0 0.0 0.0 1.0]  GraphicShininess=75  GraphicOpacity=smiData.Solid(5).opacity  GeometryShape=FromFile  RectangleSize=[1 1]  RectangleSizeUnits=m  BrickDimensions=[1 1 1]  BrickDimensionUnits=m  CylinderRadius=1  CylinderRadiusUnits=m  CylinderLength=1  CylinderLengthUnits=m  SphereRadius=1  SphereRadiusUnits=m  EllipsoidRadii=[1 1 1]  EllipsoidRadiiUnits=m  ExtrusionCrossSection=[1 1; -1 1; -1 -1; 1 -1]  ExtrusionCrossSectionUnits=m  ExtrusionLength=1  ExtrusionLengthUnits=m  PolygonNumSides=3  PolygonOuterRadius=1  PolygonOuterRadiusUnits=m  ExtGeomFileType=STEP  ExtGeomFileName=Part6_Default_sldprt.STEP  ExtGeomFileUnits=m  RevolutionCrossSection=[1 1; 1 -1; 2 -1; 2 1]  RevolutionCrossSectionUnits=m  RevolutionExtent=Full  RevolutionAngle=180  RevolutionAngleUnits=deg
  Transform : sm_lib/Frames and Transforms/Rigid Transform  TranslationMethod=Cartesian  TranslationStandardOffset=0  TranslationLengthUnit=mm  TranslationStandardAxis=+Z  TranslationCartesianOffset=smiData.RigidTransform(10).translation  TranslationROffset=0  TranslationROffsetUnits=m  TranslationZOffset=0  TranslationZOffsetUnits=m  TranslationThetaOffset=0  TranslationThetaOffsetUnits=deg  RotationMethod=ArbitraryAxis  RotationAngleUnits=rad  RotationStandardAxis=+Z  RotationAngle=smiData.RigidTransform(10).angle  RotationArbitraryAxis=smiData.RigidTransform(10).axis  FollAlignAxisA=+X  BaseAlignAxisA=+Y  FollAlignAxisB=+Y  BaseAlignAxisB=+Z  RotationSequenceAxes=FollowerAxes  RotationSequence=XYX  RotationSequenceAngles=[0 0 0]  RotationSequenceAnglesUnits=deg  RotationMatrix=[1 0 0; 0 1 0; 0 0 1]
  F : PMIOPort  Port=1  Side=Left
  connections:
  Solid/RConn1 -- ReferenceFrame/RConn1 -- Transform/LConn1
  Transform/RConn1 -- F/RConn1

== matlab function Assem1/Inverse Kinematics ==
  data: P_EE_x input; P_EE_y input; P_EE_z input; the1 output; phi input; the2 output; the3 output; the4 output
function [the1,the2,the3,the4]=IK_4DOF(P_EE_x,P_EE_y,P_EE_z,phi)
l1=150; l2=350; l3=363.5; l4=210;
d1=140;
 % tim the1
the1=atan2d(P_EE_y,P_EE_x);
Px=P_EE_x-l4*cosd(the1)*cosd(phi);
Py=P_EE_y-l4*sind(the1)*cosd(phi);
Pz=P_EE_z+l4*sind(phi);

 %tim theta3 >0
 nx=Px*cosd(the1)+Py*sind(the1)-l1;
 ny=Pz-d1;
 c3=(nx*nx+ny*ny-l3*l3-l2*l2)/(2*l2*l3);
 s3=sqrt(1-c3^2);
 the3=atan2d(s3,c3);
 %tim theta2 >0;
 the2=atan2d(-((ny*(l3*cosd(the3)+l2)+l3*sind(the3)*nx)),-((-nx*(l3*cosd(the3)+l2)+l3*sind(the3)*ny)));
 %tim theta4 
 the4=phi-the2-the3;

== matlab function Assem1/Forward Kinematics ==
  data: the1 input; P_EE_X output; the2 input; the3 input; the4 input; P_EE_Y output; P_EE_Z output
function [P_EE_X,P_EE_Y,P_EE_Z]=FK_4DOF(the1,the2,the3,the4)
l1=150; l2=350; l3=363.5; l4=210;
d1=140;
P_EE_X=cosd(the1)*(l1+l3*cosd(the2+the3)+l2*cosd(the2)+l4*cosd(the2+the3+the4));
P_EE_Y=sind(the1)*(l1+l3*cosd(the2+the3)+l2*cosd(the2)+l4*cosd(the2+the3+the4));
P_EE_Z=d1-l3*sind(the2+the3)-l2*sind(the2)-l4*sind(the2+the3+the4);
end

== matlab function Assem1/Subsystem/LINE    ==
  data: x output; t input; y output; P0 input; v0 input; Pf input; vf input; tf input; z output
function [x,y,z] = LINE(t,P0,v0,Pf,vf,tf)
a10=P0(1);
a20=P0(2);
a30=P0(3);
a11=v0(1);
a21=v0(2);
a31=v0(3);
a12=3/tf^2*(Pf(1)-P0(1))-2/tf*v0(1)-1/tf*vf(1);
a22=3/tf^2*(Pf(2)-P0(2))-2/tf*v0(2)-1/tf*vf(2);
a32=3/tf^2*(Pf(3)-P0(3))-2/tf*v0(3)-1/tf*vf(3);
a13=-2/tf^3*(Pf(1)-P0(1))+1/tf^2*(vf(1)+v0(1));
a23=-2/tf^3*(Pf(2)-P0(2))+1/tf^2*(vf(2)+v0(2));
a33=-2/tf^3*(Pf(3)-P0(3))+1/tf^2*(vf(3)+v0(3));
if t<30
    x=a10+a11*t+a12*t^2+a13*t^3;
    y=a20+a21*t+a22*t^2+a23*t^3;
    z=a30+a31*t+a32*t^2+a33*t^3; 
else
    t=30;
    x=a10+a11*t+a12*t^2+a13*t^3;
    y=a20+a21*t+a22*t^2+a23*t^3;
    z=a30+a31*t+a32*t^2+a33*t^3; 
end

== matlab function Assem1/Subsystem/Triangle ==
  data: x output; t input; y output; p input; z output
function [x,y,z] = Triangle(t,p)
t0=0;
tf=10;
t1=t;
v0=0;
vf=0;
%Phương trình quĩ đạo bậc 3: P(t) = a0 + a1*t+ a2*t^2 + a3*t^3
A=[ 1 t0 t0^2 t0^3;
    0  1  2*t0 3*t0^2; 
    1 tf tf^2 tf^3;
    0 1  2*tf 3*tf^2;];
if t<=10
%%
C=[ p(1,1); v0; p(2,1); vf];
Bx=A\C;
x = Bx(1,1) + Bx(2,1)*t1 +Bx(3,1)*t1^2 + Bx(4,1)*t1^3;
C=[p(1,2); v0; p(2,2); vf];
By=A\C;
y = By(1,1) + By(2,1)*t1 +By(3,1)*t1^2 + By(4,1)*t1^3;
C=[p(1,3); v0; p(2,3); vf];
Bz=A\C;
z = Bz(1,1) + Bz(2,1)*t1 +Bz(3,1)*t1^2 + Bz(4,1)*t1^3;
elseif (t>10)&&(t<=20)
t1=t1-10;
C=[ p(2,1); v0; p(3,1); vf];
Bx=A\C;
x = Bx(1,1) + Bx(2,1)*t1 +Bx(3,1)*t1^2 + Bx(4,1)*t1^3;
C=[ p(2,2); v0; p(3,2); vf];
By=A\C;
y = By(1,1) + By(2,1)*t1 +By(3,1)*t1^2 + By(4,1)*t1^3;

C=[ p(2,3); v0; p(3,3); vf];
Bz=A\C;
z = Bz(1,1) + Bz(2,1)*t1 +Bz(3,1)*t1^2 + Bz(4,1)*t1^3;
elseif t<30
t1=t1-20;
C=[p(3,1); v0; p(1,1); vf];
Bx=A\C;
x = Bx(1,1) + Bx(2,1)*t1 +Bx(3,1)*t1^2 + Bx(4,1)*t1^3;
C=[ p(3,2); v0; p(1,2); vf];
By=A\C;
y = By(1,1) + By(2,1)*t1 +By(3,1)*t1^2 + By(4,1)*t1^3;

C=[ p(3,3); v0; p(1,3); vf];
Bz=A\C;
z = Bz(1,1) + Bz(2,1)*t1 +Bz(3,1)*t1^2 + Bz(4,1)*t1^3;
else
t1=30;
t1=t1-20;
C=[p(3,1); v0; p(1,1); vf];
Bx=A\C;
x = Bx(1,1) + Bx(2,1)*t1 +Bx(3,1)*t1^2 + Bx(4,1)*t1^3;
C=[ p(3,2); v0; p(1,2); vf];
By=A\C;
y = By(1,1) + By(2,1)*t1 +By(3,1)*t1^2 + By(4,1)*t1^3;
C=[ p(3,3); v0; p(1,3); vf];
Bz=A\C;
z = Bz(1,1) + Bz(2,1)*t1 +Bz(3,1)*t1^2 + Bz(4,1)*t1^3;
end

== matlab function Assem1/Subsystem/MATLAB Function ==
  data: x output; t input; y output; p input; z output
function [x,y,z] = Rectangle(t,p)
t0=0;
tf=10;
t1=t;
v0=0;
vf=0;
%Phương trình quĩ đạo bậc 3: P(t) = a0 + a1*t+ a2*t^2 + a3*t^3
A=[ 1 t0 t0^2 t0^3;
    0  1  2*t0 3*t0^2; 
    1 tf tf^2 tf^3;
    0 1  2*tf 3*tf^2;];
if t<=10
%%
C=[ p(1,1); v0; p(2,1); vf];
Bx=A\C;
x = Bx(1,1) + Bx(2,1)*t1 +Bx(3,1)*t1^2 + Bx(4,1)*t1^3;
C=[p(1,2); v0; p(2,2); vf];
By=A\C;
y = By(1,1) + By(2,1)*t1 +By(3,1)*t1^2 + By(4,1)*t1^3;
C=[p(1,3); v0; p(2,3); vf];
Bz=A\C;
z = Bz(1,1) + Bz(2,1)*t1 +Bz(3,1)*t1^2 + Bz(4,1)*t1^3;
elseif (t>10)&&(t<=20)
t1=t1-10;
C=[ p(2,1); v0; p(3,1); vf];
Bx=A\C;
x = Bx(1,1) + Bx(2,1)*t1 +Bx(3,1)*t1^2 + Bx(4,1)*t1^3;
C=[ p(2,2); v0; p(3,2); vf];
By=A\C;
y = By(1,1) + By(2,1)*t1 +By(3,1)*t1^2 + By(4,1)*t1^3;

C=[ p(2,3); v0; p(3,3); vf];
Bz=A\C;
z = Bz(1,1) + Bz(2,1)*t1 +Bz(3,1)*t1^2 + Bz(4,1)*t1^3;
elseif (t>20)&&(t<=30) 
t1=t1-20;
C=[p(3,1); v0; p(4,1); vf];
Bx=A\C;
x = Bx(1,1) + Bx(2,1)*t1 +Bx(3,1)*t1^2 + Bx(4,1)*t1^3;
C=[ p(3,2); v0; p(4,2); vf];
By=A\C;
y = By(1,1) + By(2,1)*t1 +By(3,1)*t1^2 + By(4,1)*t1^3;

C=[ p(3,3); v0; p(4,3); vf];
Bz=A\C;
z = Bz(1,1) + Bz(2,1)*t1 +Bz(3,1)*t1^2 + Bz(4,1)*t1^3;

elseif t1<=40
t1=t1-30;
C=[p(4,1); v0; p(1,1); vf];
Bx=A\C;
x = Bx(1,1) + Bx(2,1)*t1 +Bx(3,1)*t1^2 + Bx(4,1)*t1^3;
C=[ p(4,2); v0; p(1,2); vf];
By=A\C;
y = By(1,1) + By(2,1)*t1 +By(3,1)*t1^2 + By(4,1)*t1^3;

C=[ p(4,3); v0; p(1,3); vf];
Bz=A\C;
z = Bz(1,1) + Bz(2,1)*t1 +Bz(3,1)*t1^2 + Bz(4,1)*t1^3;
else
t1=40;
t1=t1-30;
C=[p(4,1); v0; p(1,1); vf];
Bx=A\C;
x = Bx(1,1) + Bx(2,1)*t1 +Bx(3,1)*t1^2 + Bx(4,1)*t1^3;
C=[ p(4,2); v0; p(1,2); vf];
By=A\C;
y = By(1,1) + By(2,1)*t1 +By(3,1)*t1^2 + By(4,1)*t1^3;

C=[ p(4,3); v0; p(1,3); vf];
Bz=A\C;
z = Bz(1,1) + Bz(2,1)*t1 +Bz(3,1)*t1^2 + Bz(4,1)*t1^3;
end
